simulink model "model_po"  (Simulink 6.3)
settings: Solver=ode45  StartTime=0.0  StopTime=10.0  RelTol=1e-3
libraries: cstblocks x4
settings Model: Creator=fromion  LastModifiedBy=xavier.litrico  ExtModeTrigMode=oneshot  ExtModeArmWhenConnect=off  BufferReuse=off  StrictBusMsg=None
settings DataIOCC: InitialState=[]  LimitDataPoints=off  LoadInitialState=on
settings OptimizationCC: BlockReduction=off  BooleanDataType=off  InlineParams=on  BufferReuse=off
settings DebuggingCC: SolverPrmCheckMsg=none
settings HardwareCC: TargetUnknown=on

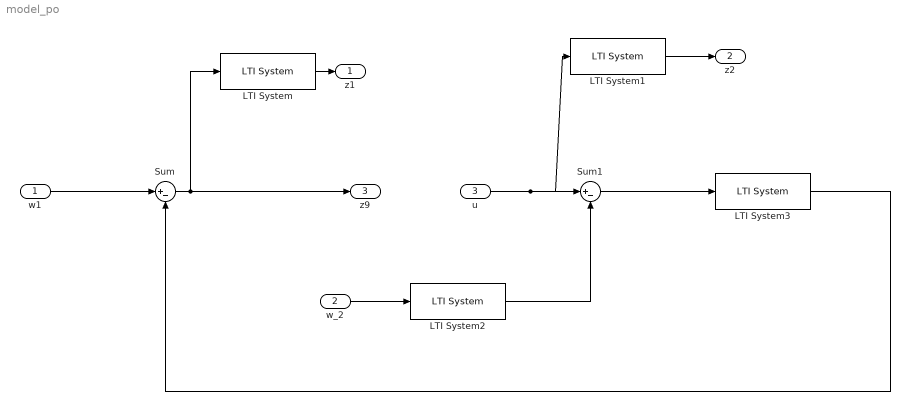
== system model_po ==
  w1 : Inport
  w_2 : Inport  Port=2
  u : Inport  Port=3
  LTI System : cstblocks/LTI System  sys=W1  IC=0
  LTI System1 : cstblocks/LTI System  sys=W2  IC=0
  LTI System2 : cstblocks/LTI System  sys=Wp  IC=0
  LTI System3 : cstblocks/LTI System  sys=sys_synt_ss  IC=0
  Sum : Sum  Inputs=|+-  SaturateOnIntegerOverflow=on  InputSameDT=on
  Sum1 : Sum  Inputs=|+-  SaturateOnIntegerOverflow=on  InputSameDT=on
  z1 : Outport
  z2 : Outport  Port=2
  z9 : Outport  Port=3
  wires:
  Sum/1 -> z9/1, LTI System/1
  LTI System1/1 -> z2/1
  w_2/1 -> LTI System2/1
  w1/1 -> Sum/1
  LTI System/1 -> z1/1
  LTI System3/1 -> Sum/2
  u/1 -> Sum1/1, LTI System1/1
  Sum1/1 -> LTI System3/1
  LTI System2/1 -> Sum1/2
